simulink model "antiWindup1"  (R2019a)
settings: Solver=VariableStepAuto  StartTime=0.0  StopTime=30  RelTol=1e-3
values from neighbouring files (symbols this model uses):
  Kp = 2    [mainAntiWindup1.m]    (also in mainAntiWindup2.m; mainBumpless.m; mainLimAzioneDerivativa.m; mainWindupIntegrale.m = 0)
  Ti = Kp/Ki    (= 1)    [mainAntiWindup1.m]    (also in mainAntiWindup2.m; mainBumpless.m; mainLimAzioneDerivativa.m = 2)
  UM = 1.05    [mainAntiWindup1.m]    (also in mainAntiWindup2.m; mainBumpless.m = inf; mainWindupIntegrale.m)
settings Model: Creator=adria  LastModifiedBy=adria

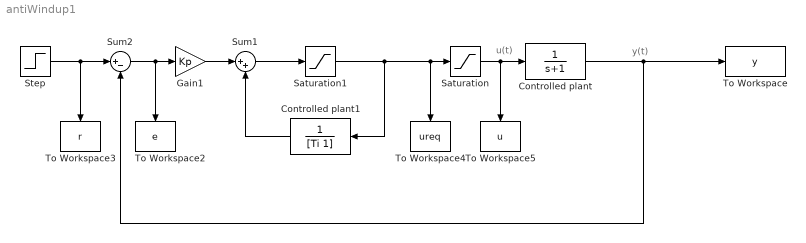
== system antiWindup1 ==
  note: u(t)
  note: y(t)
  Controlled plant : TransferFcn  Denominator=[1 1]
  Controlled plant1 : TransferFcn  Denominator=[Ti 1]
  Gain1 : Gain  Gain=Kp
  Saturation : Saturate  UpperLimit=UM  LowerLimit=-UM
  Saturation1 : Saturate  UpperLimit=UM  LowerLimit=-UM
  Step : Step  SampleTime=0
  Sum1 : Sum  Inputs=|++
  Sum2 : Sum  Inputs=|+-
  To Workspace : ToWorkspace  VariableName=y  SaveFormat=Structure With Time  SampleTime=-1
  To Workspace2 : ToWorkspace  VariableName=e  SaveFormat=Structure With Time  SampleTime=-1
  To Workspace3 : ToWorkspace  VariableName=r  SaveFormat=Structure With Time  SampleTime=-1
  To Workspace4 : ToWorkspace  VariableName=ureq  SaveFormat=Structure With Time  SampleTime=-1
  To Workspace5 : ToWorkspace  VariableName=u  SaveFormat=Structure With Time  SampleTime=-1
  wires:
  Step/1 -> To Workspace3/1, Sum2/1
  Saturation1/1 -> Controlled plant1/1, To Workspace4/1, Saturation/1
  Gain1/1 -> Sum1/1
  Controlled plant/1 -> Sum2/2, To Workspace/1
  Sum2/1 -> Gain1/1, To Workspace2/1
  Saturation/1 -> To Workspace5/1, Controlled plant/1
  Sum1/1 -> Saturation1/1
  Controlled plant1/1 -> Sum1/2
